simulink model "fuzzCont"  (R2018a)
settings: Solver=VariableStepAuto  StartTime=0.0  StopTime=10.0  RelTol=1e-3
libraries: fuzblock x1
settings Model: Creator=chows  LastModifiedBy=chows

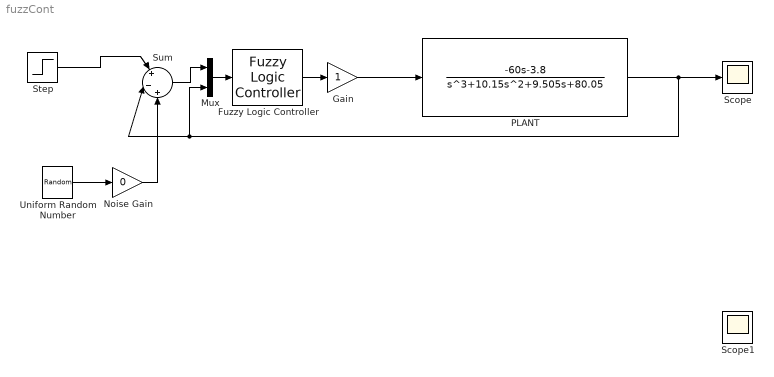
== system fuzzCont ==
  " PLANT" : TransferFcn  Numerator=[-60 -3.8]  Denominator=[1 10.15 9.505 80.05]
  Fuzzy Logic Controller : fuzblock/Fuzzy Logic  Controller  FIS=control.fis  OutputSampleNumber=101  DataType=double  FuzzifiedInputs=off  RuleFiringStrengths=off  RuleOutputs=off  AggregatedOutputs=off  SimulateUsing=Interpreted execution  OutOfRangeInputValueMessage=warning  NoRuleFiredMessage=warning  EmptyOutputFuzzySetMessage=warning
  Gain : Gain
  Mux : Mux  Inputs=2
  Noise Gain : Gain  Gain=0
  Scope : Scope
  Scope1 : Scope
  Step : Step  SampleTime=0
  Sum : Sum  Inputs=|+|-|+
  Uniform Random Number : UniformRandomNumber  SampleTime=0.1
  wires:
  Fuzzy Logic Controller/1 -> Gain/1
  Gain/1 -> " PLANT"/1
  " PLANT"/1 -> Mux/2, Sum/2, Scope/1
  Uniform Random Number/1 -> Noise Gain/1
  Noise Gain/1 -> Sum/3
  Step/1 -> Sum/1
  Mux/1 -> Fuzzy Logic Controller/1
  Sum/1 -> Mux/1
